simulink model "Scratch3"  (Simulink 8.5)
settings: Solver=ode4  StartTime=0.0  StopTime=20  FixedStep=0.005  RelTol=1e-3
model workspace (MAT data in the model file):
  Jm1 = 0.9333
  Jm2 = 0.6533
  Jm3 = 0.6533
  Jm4 = 0.4667
  k1 = 100
  k2 = 100
  k3 = 100
  k4 = 100
  Fv1 = 15
  Fv2 = 12
  Fv3 = 1
  Fv4 = 1
  Kp1 = 15
  Kp2 = 20
  Kp3 = 5
  Kp4 = 5
  Kd1 = 5
  Kd2 = 10
  Kd3 = 2
  Kd4 : num (value not decoded)
libraries: dspinverses x1, roblocks x1
(part 1 of 3)
settings Model: Creator=ahmad  LastModifiedBy=ahmad
settings DataIOCC: SignalLoggingSaveFormat=Dataset
settings OptimizationCC: ExpressionDepthLimit=128
settings DebuggingCC: UnderspecifiedInitializationDetection=Simplified  MergeDetectMultiDrivingBlocksExec=error  FcnCallInpInsideContextMsg=EnableAllAsError  StateNameClashWarn=none
settings GRTTargetCC: CombineOutputUpdateFcns=on  GRTInterface=off

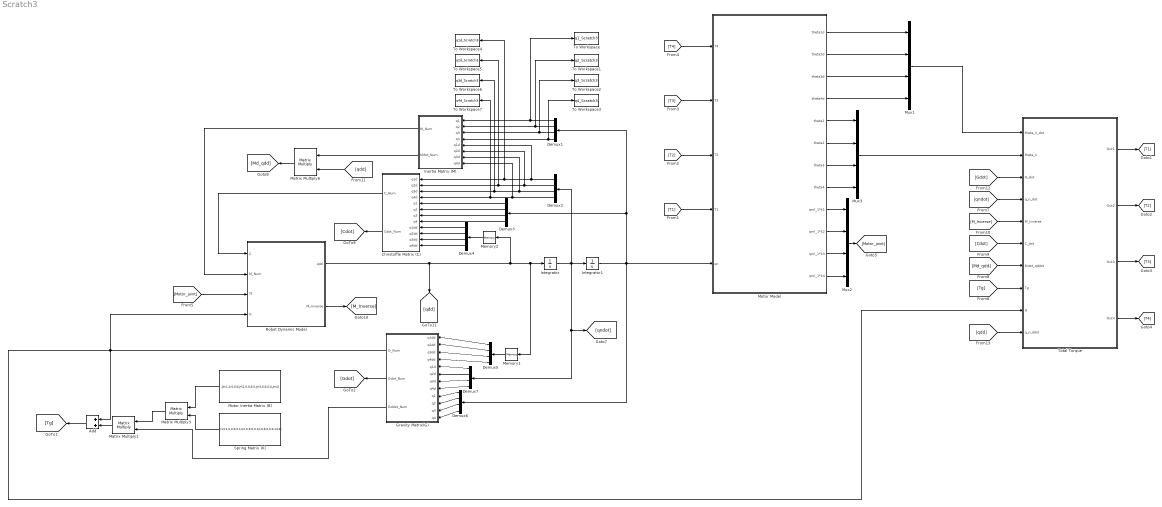
== system Scratch3 ==
  Add : Sum
  Christoffle Matrix (C) : MATLAB Function  TreatAsAtomicUnit=on
  Demux{1..7} (7 alike) : Demux
  Gravity Matrix(G) : MATLAB Function  TreatAsAtomicUnit=on
  Inertia Matrix (M) : MATLAB Function  TreatAsAtomicUnit=on
  Integrator : Integrator
  Integrator1 : Integrator
  Matrix Multiply1 : Product  Multiplication=Matrix(*)
  Matrix Multiply3 : Product  Multiplication=Matrix(*)
  Matrix Multiply6 : Product  Multiplication=Matrix(*)
  Memory1 : Memory
  Memory2 : Memory
  Motor Inertia Matrix (B) : Constant  Value=[Jm1,0,0,0;0,Jm2,0,0;0,0,Jm3,0;0,0,0,Jm4]  VectorParams1D=off
  "Motor Model " : Subsystem
  Mux1 : Mux
  Mux2 : Mux
  Mux3 : Mux
  "Robot Dynamic Model " : MATLAB Function  TreatAsAtomicUnit=on
  Spring Matrix (K) : Constant  Value=[1/k1,0,0,0;0,1/k2,0,0;0,0,1/k3,0;0,0,0,1/k4]  VectorParams1D=off
  To Workspace : ToWorkspace  VariableName=q1_Scratch3  SaveFormat=Structure With Time  SampleTime=-1
  To Workspace1 : ToWorkspace  VariableName=q2_Scratch3  SaveFormat=Structure With Time  SampleTime=-1
  To Workspace2 : ToWorkspace  VariableName=q3_Scratch3  SaveFormat=Structure With Time  SampleTime=-1
  To Workspace3 : ToWorkspace  VariableName=q4_Scratch3  SaveFormat=Structure With Time  SampleTime=-1
  To Workspace4 : ToWorkspace  VariableName=q1d_Scratch3  SaveFormat=Structure With Time  SampleTime=-1
  To Workspace5 : ToWorkspace  VariableName=q2d_Scratch3  SaveFormat=Structure With Time  SampleTime=-1
  To Workspace6 : ToWorkspace  VariableName=q3d_Scratch3  SaveFormat=Structure With Time  SampleTime=-1
  To Workspace7 : ToWorkspace  VariableName=q4d_Scratch3  SaveFormat=Structure With Time  SampleTime=-1
  "Total Torque " : Subsystem
  wires:
  [T1] -> "Motor Model "/4(T1)
  [T2] -> "Motor Model "/3(T2)
  [T3] -> "Motor Model "/2(T3)
  [T4] -> "Motor Model "/1(T4)
  "Motor Model "/9(qml_1*k1) -> Mux2/1
  "Motor Model "/10(qml_1*k2) -> Mux2/2
  "Motor Model "/11(qml_1*k3) -> Mux2/3
  "Motor Model "/12(qml_1*k4) -> Mux2/4
  Mux2/1 -> [Motor_joint]
  "Total Torque "/4(Out4) -> [T4]
  "Total Torque "/3(Out3) -> [T3]
  "Total Torque "/2(Out2) -> [T2]
  "Total Torque "/1(Out1) -> [T1]
  "Motor Model "/1(theta1d) -> Mux1/1
  "Motor Model "/2(theta2d) -> Mux1/2
  "Motor Model "/3(theta3d) -> Mux1/3
  "Motor Model "/4(theta4d) -> Mux1/4
  Integrator/1 -> Demux7/1, [qndot], Demux2/1, Integrator1/1
  Integrator1/1 -> Demux1/1, Demux3/1, "Motor Model "/5(qn), Demux6/1
  Demux2/1 -> Inertia Matrix (M)/5(q1d), To Workspace4/1, Christoffle Matrix (C)/1(q1d)
  Demux2/2 -> Inertia Matrix (M)/6(q2d), To Workspace5/1, Christoffle Matrix (C)/2(q2d)
  Demux2/3 -> Inertia Matrix (M)/7(q3d), To Workspace6/1, Christoffle Matrix (C)/3(q3d)
  Demux2/4 -> Inertia Matrix (M)/8(q4d), Christoffle Matrix (C)/4(q4d), To Workspace7/1
  Demux3/1 -> Christoffle Matrix (C)/5(q1)
  Demux3/2 -> Christoffle Matrix (C)/6(q2)
  Demux3/3 -> Christoffle Matrix (C)/7(q3)
  Demux3/4 -> Christoffle Matrix (C)/8(q4)
  Demux1/1 -> Inertia Matrix (M)/1(q1), To Workspace/1
  Demux1/2 -> Inertia Matrix (M)/2(q2), To Workspace1/1
  Demux1/3 -> Inertia Matrix (M)/3(q3), To Workspace2/1
  Demux1/4 -> Inertia Matrix (M)/4(q4), To Workspace3/1
  Demux4/1 -> Christoffle Matrix (C)/9(q1dd)
  Demux4/2 -> Christoffle Matrix (C)/10(q2dd)
  Demux4/3 -> Christoffle Matrix (C)/11(q3dd)
  Demux4/4 -> Christoffle Matrix (C)/12(q4dd)
  Christoffle Matrix (C)/2(Cdot_Num) -> [Cdot]
  [qdd] -> Matrix Multiply6/2
  Matrix Multiply6/1 -> [Md_qdd]
  "Robot Dynamic Model "/2(M_Inverse) -> [M_Inverse]
  [M_Inverse] -> "Total Torque "/5(M_Inverse)
  [Md_qdd] -> "Total Torque "/7(Mdot_qddot)
  [Cdot] -> "Total Torque "/6(C_dot)
  [qndot] -> "Total Torque "/4(q_n_dot)
  "Robot Dynamic Model "/1(qdd) -> [qdd], Memory1/1, Integrator/1, Memory2/1
  Inertia Matrix (M)/2(Mdot_Num) -> Matrix Multiply6/1
  [Tg] -> "Total Torque "/8(Tg)
  Motor Inertia Matrix (B)/1 -> Matrix Multiply3/1
  Spring Matrix (K)/1 -> Matrix Multiply3/2
  Matrix Multiply3/1 -> Matrix Multiply1/1
  Demux6/1 -> Gravity Matrix(G)/9(q1)
  Demux6/2 -> Gravity Matrix(G)/10(q2)
  Demux6/3 -> Gravity Matrix(G)/11(q3)
  Demux6/4 -> Gravity Matrix(G)/12(q4)
  Demux5/1 -> Gravity Matrix(G)/1(q1dd)
  Demux5/2 -> Gravity Matrix(G)/2(q2dd)
  Demux5/3 -> Gravity Matrix(G)/3(q3dd)
  Demux5/4 -> Gravity Matrix(G)/4(q4dd)
  Demux7/1 -> Gravity Matrix(G)/5(q1d)
  Demux7/2 -> Gravity Matrix(G)/6(q2d)
  Demux7/3 -> Gravity Matrix(G)/7(q3d)
  Demux7/4 -> Gravity Matrix(G)/8(q4d)
  Add/1 -> [Tg]
  Matrix Multiply1/1 -> Add/2
  [Gdot] -> "Total Torque "/3(G_dot)
  "Motor Model "/8(theta4) -> Mux3/4
  "Motor Model "/7(theta3) -> Mux3/3
  "Motor Model "/6(theta2) -> Mux3/2
  "Motor Model "/5(theta1) -> Mux3/1
  Mux3/1 -> "Total Torque "/2(theta_n)
  Mux1/1 -> "Total Torque "/1(theta_n_dot)
  Christoffle Matrix (C)/1(C_Num) -> "Robot Dynamic Model "/1(C)
  [Motor_joint] -> "Robot Dynamic Model "/3(Tf)
  Inertia Matrix (M)/1(M_Num) -> "Robot Dynamic Model "/2(M_Num)
  [qdd] -> "Total Torque "/10("q_n_ddot ")
  Gravity Matrix(G)/1(G_Num) -> "Robot Dynamic Model "/4(G), "Total Torque "/9(G), Add/1
  Memory2/1 -> Demux4/1
  Memory1/1 -> Demux5/1
  Gravity Matrix(G)/3(Gddot_Num) -> Matrix Multiply1/2
  Gravity Matrix(G)/2(Gdot_Num) -> [Gdot]

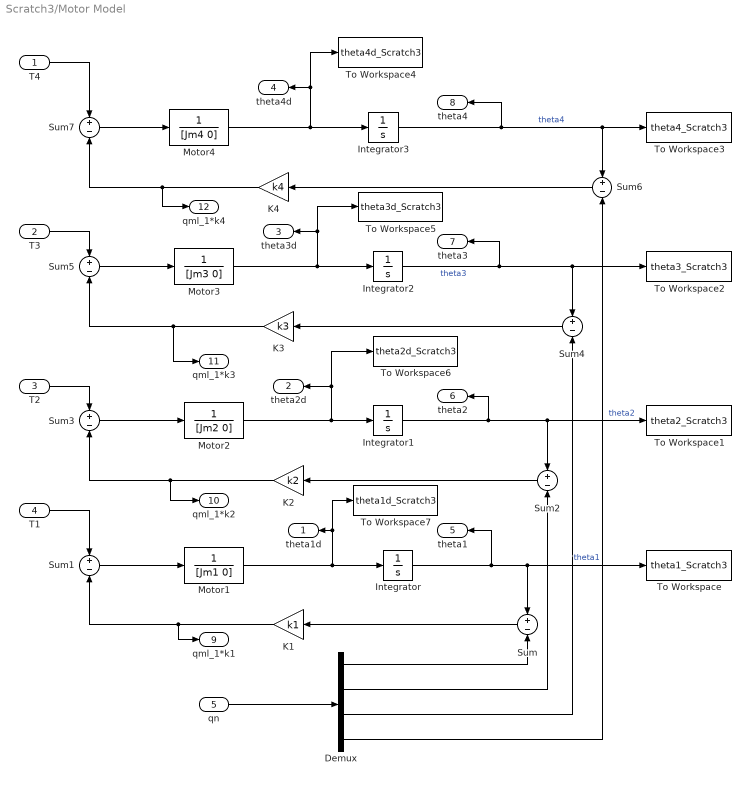
== system Scratch3/Motor Model  ==
  T4 : Inport
  T3 : Inport  Port=2
  T2 : Inport  Port=3
  T1 : Inport  Port=4
  qn : Inport  Port=5
  "\tK1 " : Gain  Gain=k1
  "\tK2 " : Gain  Gain=k2
  "\tK3 " : Gain  Gain=k3
  "\tK4 " : Gain  Gain=k4
  Demux : Demux
  Integrator{,1..3} (4 alike) : Integrator
  Motor1 : TransferFcn  Denominator=[Jm1 0]
  Motor2 : TransferFcn  Denominator=[Jm2 0]
  Motor3 : TransferFcn  Denominator=[Jm3 0]
  Motor4 : TransferFcn  Denominator=[Jm4 0]
  Sum{,1..7} (8 alike) : Sum  Inputs=+-
  To Workspace : ToWorkspace  VariableName=theta1_Scratch3  SaveFormat=Structure With Time  SampleTime=-1
  To Workspace1 : ToWorkspace  VariableName=theta2_Scratch3  SaveFormat=Structure With Time  SampleTime=-1
  To Workspace2 : ToWorkspace  VariableName=theta3_Scratch3  SaveFormat=Structure With Time  SampleTime=-1
  To Workspace3 : ToWorkspace  VariableName=theta4_Scratch3  SaveFormat=Structure With Time  SampleTime=-1
  To Workspace4 : ToWorkspace  VariableName=theta4d_Scratch3  SaveFormat=Structure With Time  SampleTime=-1
  To Workspace5 : ToWorkspace  VariableName=theta3d_Scratch3  SaveFormat=Structure With Time  SampleTime=-1
  To Workspace6 : ToWorkspace  VariableName=theta2d_Scratch3  SaveFormat=Structure With Time  SampleTime=-1
  To Workspace7 : ToWorkspace  VariableName=theta1d_Scratch3  SaveFormat=Structure With Time  SampleTime=-1
  theta1d : Outport
  theta2d : Outport  Port=2
  theta3d : Outport  Port=3
  theta4d : Outport  Port=4
  theta1 : Outport  Port=5
  theta2 : Outport  Port=6
  theta3 : Outport  Port=7
  theta4 : Outport  Port=8
  qml_1*k1 : Outport  Port=9
  qml_1*k2 : Outport  Port=10
  qml_1*k3 : Outport  Port=11
  qml_1*k4 : Outport  Port=12
  wires:
  qn/1 -> Demux/1
  Demux/1 -> Sum/2
  Motor1/1 -> Integrator/1, To Workspace7/1, theta1d/1
  Integrator/1 -> theta1/1, To Workspace/1, Sum/1  "theta1"
  Sum/1 -> "\tK1 "/1
  "\tK1 "/1 -> Sum1/2, qml_1*k1/1
  Sum1/1 -> Motor1/1
  Motor2/1 -> To Workspace6/1, theta2d/1, Integrator1/1
  Integrator1/1 -> theta2/1, To Workspace1/1, Sum2/1  "theta2"
  Sum2/1 -> "\tK2 "/1
  "\tK2 "/1 -> qml_1*k2/1, Sum3/2
  Sum3/1 -> Motor2/1
  Demux/2 -> Sum2/2
  Motor3/1 -> To Workspace5/1, theta3d/1, Integrator2/1
  Integrator2/1 -> theta3/1, To Workspace2/1, Sum4/1  "theta3"
  Sum4/1 -> "\tK3 "/1
  "\tK3 "/1 -> qml_1*k3/1, Sum5/2
  Sum5/1 -> Motor3/1
  Demux/3 -> Sum4/2
  Motor4/1 -> To Workspace4/1, theta4d/1, Integrator3/1
  Integrator3/1 -> theta4/1, To Workspace3/1, Sum6/1  "theta4"
  Sum6/1 -> "\tK4 "/1
  "\tK4 "/1 -> qml_1*k4/1, Sum7/2
  Sum7/1 -> Motor4/1
  Demux/4 -> Sum6/2
  T4/1 -> Sum7/1
  T3/1 -> Sum5/1
  T2/1 -> Sum3/1
  T1/1 -> Sum1/1

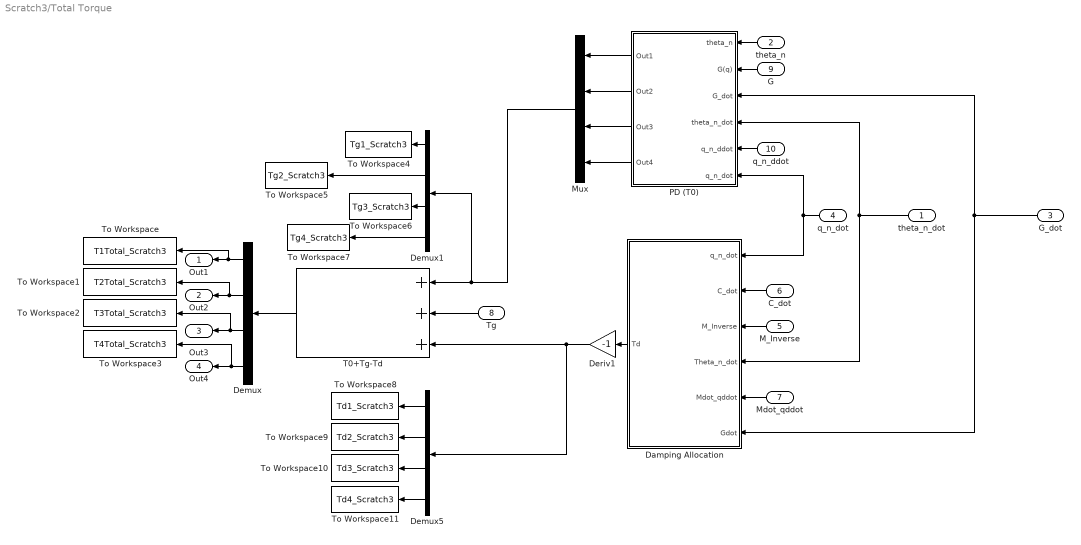
== system Scratch3/Total Torque  ==
  theta_n_dot : Inport
  theta_n : Inport  Port=2
  G_dot : Inport  Port=3
  q_n_dot : Inport  Port=4
  M_Inverse : Inport  Port=5
  C_dot : Inport  Port=6
  Mdot_qddot : Inport  Port=7
  Tg : Inport  Port=8
  G : Inport  Port=9
  "q_n_ddot " : Inport  Port=10
  Damping Allocation : Subsystem
  Demux : Demux
  Demux1 : Demux
  Demux5 : Demux
  Deriv1 : Gain  Gain=-1
  Mux : Mux
  PD (T0) : Subsystem
  T0+Tg-Td : Sum  Inputs=+++
  To Workspace : ToWorkspace  VariableName=T1Total_Scratch3  SaveFormat=Structure With Time  SampleTime=-1
  To Workspace1 : ToWorkspace  VariableName=T2Total_Scratch3  SaveFormat=Structure With Time  SampleTime=-1
  To Workspace10 : ToWorkspace  VariableName=Td3_Scratch3  SaveFormat=Structure With Time  SampleTime=-1
  To Workspace11 : ToWorkspace  VariableName=Td4_Scratch3  SaveFormat=Structure With Time  SampleTime=-1
  To Workspace2 : ToWorkspace  VariableName=T3Total_Scratch3  SaveFormat=Structure With Time  SampleTime=-1
  To Workspace3 : ToWorkspace  VariableName=T4Total_Scratch3  SaveFormat=Structure With Time  SampleTime=-1
  To Workspace4 : ToWorkspace  VariableName=Tg1_Scratch3  SaveFormat=Structure With Time  SampleTime=-1
  To Workspace5 : ToWorkspace  VariableName=Tg2_Scratch3  SaveFormat=Structure With Time  SampleTime=-1
  To Workspace6 : ToWorkspace  VariableName=Tg3_Scratch3  SaveFormat=Structure With Time  SampleTime=-1
  To Workspace7 : ToWorkspace  VariableName=Tg4_Scratch3  SaveFormat=Structure With Time  SampleTime=-1
  To Workspace8 : ToWorkspace  VariableName=Td1_Scratch3  SaveFormat=Structure With Time  SampleTime=-1
  To Workspace9 : ToWorkspace  VariableName=Td2_Scratch3  SaveFormat=Structure With Time  SampleTime=-1
  Out1 : Outport
  Out2 : Outport  Port=2
  Out3 : Outport  Port=3
  Out4 : Outport  Port=4
  wires:
  PD (T0)/1(Out1) -> Mux/1
  PD (T0)/2(Out2) -> Mux/2
  PD (T0)/3(Out3) -> Mux/3
  PD (T0)/4(Out4) -> Mux/4
  T0+Tg-Td/1 -> Demux/1
  Demux/2 -> To Workspace1/1, Out2/1
  Demux/3 -> To Workspace2/1, Out3/1
  Demux/4 -> To Workspace3/1, Out4/1
  Tg/1 -> T0+Tg-Td/2
  Damping Allocation/1(Td) -> Deriv1/1
  C_dot/1 -> Damping Allocation/2(C_dot)
  M_Inverse/1 -> Damping Allocation/3(M_Inverse)
  q_n_dot/1 -> Damping Allocation/1(q_n_dot), PD (T0)/6(q_n_dot)
  Mdot_qddot/1 -> Damping Allocation/5(Mdot_qddot)
  G_dot/1 -> Damping Allocation/6(Gdot), PD (T0)/3("G_dot ")
  theta_n/1 -> PD (T0)/1(theta_n)
  G/1 -> PD (T0)/2("G(q) ")
  Mux/1 -> Demux1/1, T0+Tg-Td/1
  "q_n_ddot "/1 -> PD (T0)/5(q_n_ddot)
  theta_n_dot/1 -> PD (T0)/4(theta_n_dot), Damping Allocation/4(Theta_n_dot)
  Demux/1 -> To Workspace/1, Out1/1
  Demux1/2 -> To Workspace5/1
  Demux1/1 -> To Workspace4/1
  Demux1/3 -> To Workspace6/1
  Demux1/4 -> To Workspace7/1
  Demux5/1 -> To Workspace8/1
  Demux5/2 -> To Workspace9/1
  Demux5/3 -> To Workspace10/1
  Demux5/4 -> To Workspace11/1
  Deriv1/1 -> Demux5/1, T0+Tg-Td/3

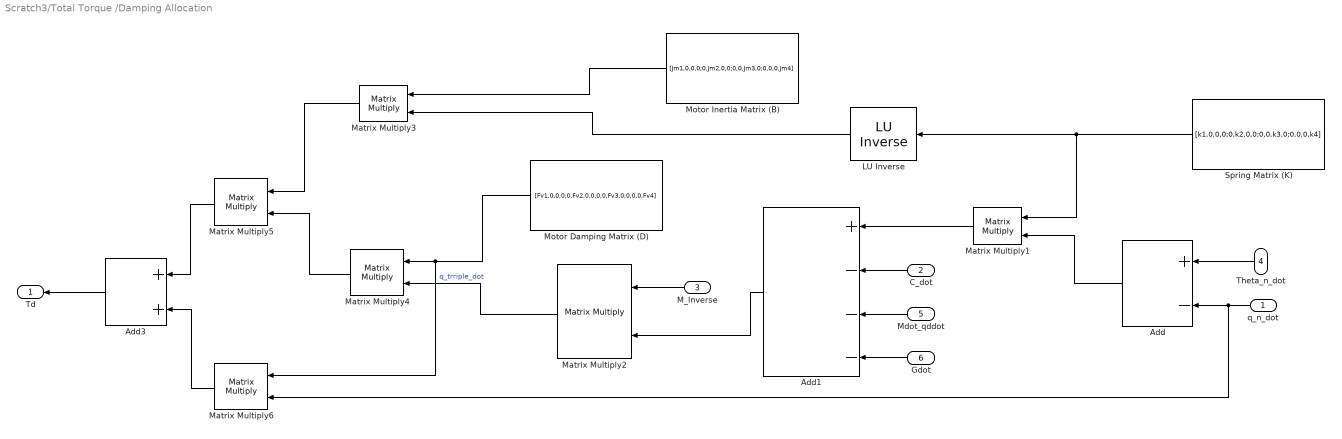
== system Scratch3/Total Torque /Damping Allocation ==
  q_n_dot : Inport
  C_dot : Inport  Port=2
  M_Inverse : Inport  Port=3
  Theta_n_dot : Inport  Port=4
  Mdot_qddot : Inport  Port=5
  Gdot : Inport  Port=6
  " LU Inverse" : dspinverses/ LU Inverse
  Add : Sum  Inputs=+-
  Add1 : Sum  Inputs=+---
  Add3 : Sum
  Matrix Multiply{1..6} (6 alike) : Product  Multiplication=Matrix(*)
  Motor Damping Matrix (D) : Constant  Value=[Fv1,0,0,0;0,Fv2,0,0;0,0,Fv3,0;0,0,0,Fv4]  VectorParams1D=off
  Motor Inertia Matrix (B) : Constant  Value=[Jm1,0,0,0;0,Jm2,0,0;0,0,Jm3,0;0,0,0,Jm4]  VectorParams1D=off
  Spring Matrix (K) : Constant  Value=[k1,0,0,0;0,k2,0,0;0,0,k3,0;0,0,0,k4]  VectorParams1D=off
  Td : Outport
  wires:
  Matrix Multiply5/1 -> Add3/1
  Matrix Multiply6/1 -> Add3/2
  q_n_dot/1 -> Matrix Multiply6/2, Add/2
  Spring Matrix (K)/1 -> Matrix Multiply1/1, " LU Inverse"/1
  Add/1 -> Matrix Multiply1/2
  Matrix Multiply1/1 -> Add1/1
  Add1/1 -> Matrix Multiply2/2
  Matrix Multiply2/1 -> Matrix Multiply4/2  "q_trriple_dot"
  Matrix Multiply4/1 -> Matrix Multiply5/2
  Motor Inertia Matrix (B)/1 -> Matrix Multiply3/1
  " LU Inverse"/1 -> Matrix Multiply3/2
  Motor Damping Matrix (D)/1 -> Matrix Multiply6/1, Matrix Multiply4/1
  Matrix Multiply3/1 -> Matrix Multiply5/1
  M_Inverse/1 -> Matrix Multiply2/1
  C_dot/1 -> Add1/2
  Mdot_qddot/1 -> Add1/3
  Add3/1 -> Td/1
  Theta_n_dot/1 -> Add/1
  Gdot/1 -> Add1/4

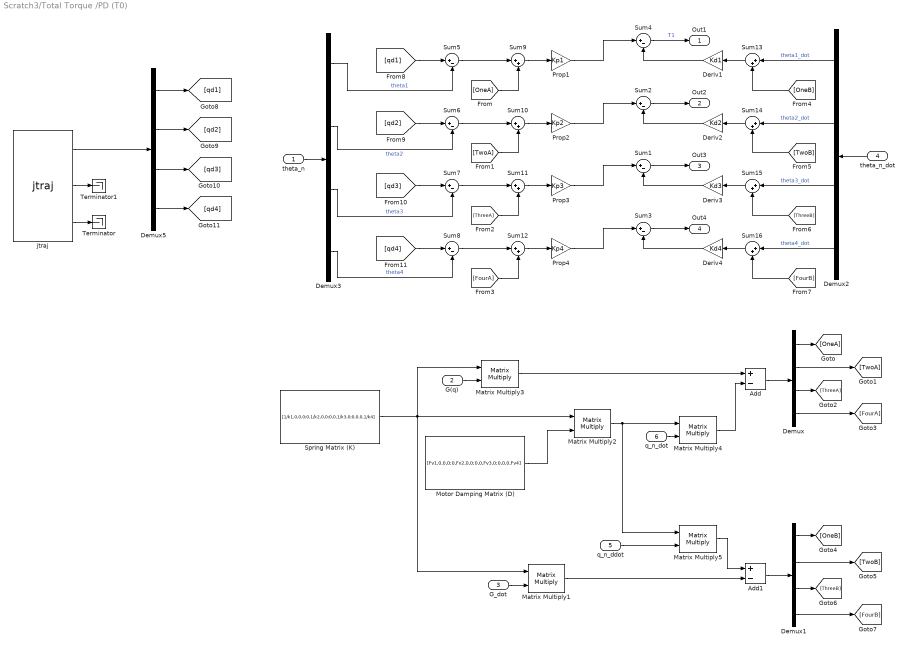
== system Scratch3/Total Torque /PD (T0) ==
  theta_n : Inport
  "G(q) " : Inport  Port=2
  "G_dot " : Inport  Port=3
  theta_n_dot : Inport  Port=4
  q_n_ddot : Inport  Port=5
  q_n_dot : Inport  Port=6
  Add : Sum  Inputs=+-
  Add1 : Sum  Inputs=+-
  Demux{,1..3,5} (5 alike) : Demux
  Deriv1 : Gain  Gain=Kd1
  Deriv2 : Gain  Gain=Kd2
  Deriv3 : Gain  Gain=Kd3
  Deriv4 : Gain  Gain=Kd4
  Matrix Multiply{1..5} (5 alike) : Product  Multiplication=Matrix(*)
  Motor Damping Matrix (D) : Constant  Value=[Fv1,0,0,0;0,Fv2,0,0;0,0,Fv3,0;0,0,0,Fv4]  VectorParams1D=off
  Prop1 : Gain  Gain=Kp1
  Prop2 : Gain  Gain=Kp2
  Prop3 : Gain  Gain=Kp3
  Prop4 : Gain  Gain=Kp4
  Spring Matrix (K) : Constant  Value=[1/k1,0,0,0;0,1/k2,0,0;0,0,1/k3,0;0,0,0,1/k4]  VectorParams1D=off
  Sum{1..8} (8 alike) : Sum  Inputs=|+-  SaturateOnIntegerOverflow=on  InputSameDT=on  OutDataTypeStr=Inherit: Same as first input
  Sum{9..16} (8 alike) : Sum  Inputs=|++  SaturateOnIntegerOverflow=on  InputSameDT=on  OutDataTypeStr=Inherit: Same as first input
  Terminator : Terminator
  Terminator1 : Terminator
  jtraj : roblocks/Trajectory/jtraj  q0=[0 0 0 0]  qf=[pi/2 -pi/2 pi/4 3*pi/2]  tmax=20  ts=0.005
  Out1 : Outport
  Out2 : Outport  Port=2
  Out3 : Outport  Port=3
  Out4 : Outport  Port=4
  wires:
  Sum4/1 -> Out1/1  "T1"
  Demux3/4 -> Sum8/2  "theta4"
  Demux2/2 -> Sum14/1  "theta2_dot"
  Demux2/3 -> Sum15/1  "theta3_dot"
  Demux2/4 -> Sum16/1  "theta4_dot"
  Demux2/1 -> Sum13/1  "theta1_dot"
  Sum3/1 -> Out4/1
  Sum1/1 -> Out3/1
  Sum2/1 -> Out2/1
  theta_n_dot/1 -> Demux2/1
  theta_n/1 -> Demux3/1
  Demux3/1 -> Sum5/2  "theta1"
  Demux3/2 -> Sum6/2  "theta2"
  Demux3/3 -> Sum7/2  "theta3"
  Sum9/1 -> Prop1/1
  Sum11/1 -> Prop3/1
  Sum12/1 -> Prop4/1
  Sum10/1 -> Prop2/1
  Spring Matrix (K)/1 -> Matrix Multiply2/1, Matrix Multiply1/1, Matrix Multiply3/1
  "G_dot "/1 -> Matrix Multiply1/2
  "G(q) "/1 -> Matrix Multiply3/2
  Sum5/1 -> Sum9/1
  [OneA] -> Sum9/2
  Sum6/1 -> Sum10/1
  Sum7/1 -> Sum11/1
  Sum8/1 -> Sum12/1
  [TwoA] -> Sum10/2
  [ThreeA] -> Sum11/2
  [FourA] -> Sum12/2
  [OneB] -> Sum13/2
  [TwoB] -> Sum14/2
  [ThreeB] -> Sum15/2
  [FourB] -> Sum16/2
  Sum16/1 -> Deriv4/1
  Sum15/1 -> Deriv3/1
  Sum14/1 -> Deriv2/1
  Sum13/1 -> Deriv1/1
  Deriv1/1 -> Sum4/2
  Deriv2/1 -> Sum2/2
  Deriv3/1 -> Sum1/2
  Deriv4/1 -> Sum3/2
  Prop4/1 -> Sum3/1
  Prop3/1 -> Sum1/1
  Prop2/1 -> Sum2/1
  Prop1/1 -> Sum4/1
  Add/1 -> Demux/1
  Demux/1 -> [OneA]
  Demux/3 -> [ThreeA]
  Demux/2 -> [TwoA]
  Demux/4 -> [FourA]
  Matrix Multiply3/1 -> Add/1
  Motor Damping Matrix (D)/1 -> Matrix Multiply2/2
  Matrix Multiply2/1 -> Matrix Multiply4/1, Matrix Multiply5/1
  q_n_dot/1 -> Matrix Multiply4/2
  Matrix Multiply4/1 -> Add/2
  Add1/1 -> Demux1/1
  Demux1/1 -> [OneB]
  Demux1/2 -> [TwoB]
  Demux1/3 -> [ThreeB]
  Demux1/4 -> [FourB]
  Matrix Multiply1/1 -> Add1/2
  q_n_ddot/1 -> Matrix Multiply5/2
  Matrix Multiply5/1 -> Add1/1
  jtraj/3 -> Terminator/1
  jtraj/2 -> Terminator1/1
  jtraj/1 -> Demux5/1
  Demux5/1 -> [qd1]
  Demux5/2 -> [qd2]
  Demux5/3 -> [qd3]
  Demux5/4 -> [qd4]
  [qd1] -> Sum5/1
  [qd2] -> Sum6/1
  [qd3] -> Sum7/1
  [qd4] -> Sum8/1

== matlab function Inertia Matrix (M) ==
  data: M_Num output double; Mdot_Num output double; q1 input double; q2 input double; q3 input double; q4 input double; q1d input double; q2d input double; q3d input double; q4d input double
function [M_Num,Mdot_Num]  = fcn(q1, q2, q3, q4, q1d, q2d, q3d, q4d)
%#codegen
% coder.extrinsic('evalin'); 
% coder.extrinsic('subs'); 
% coder.extrinsic('eval'); 
% 
% qsym = evalin('base','q');
% Msym = evalin('base','M');
% StatesSym = evalin('base','states1');
% MdotSym = evalin('base','Mdot');
% 
% q_Num= [q1t;q2t;q3t;q4t];
% States_Num = [q1t;q2t;q3t;q4t;q1dt;q2dt;q3dt;q4dt];
% 
% M_Num = zeros(4,4);
% Mdot_Num = zeros(4,4);
% 
% M_Num = eval(subs(Msym,qsym,q_Num));
% Mdot_Num = eval(subs(MdotSym,StatesSym,States_Num));

m1 = 10;
m2 = 7;
m3 = 7;
m4 = 5;
l1 = 1;
l2 = 0.7;
l3 = 0.7; 
l4 = 0.5;
d1 = l1/2;
d2 = l2/2;
d3 = l3/2; 
d4 = l4/2;
I1zz = 0.9333;
I2zz = 0.6533;
I3zz = 0.6533;
I4zz = 0.4667;

M_Num = [I1zz + I2zz + I3zz + I4zz + d1^2*m1 + (d2^2*m2)/2 + d3^2*m3 + d4^2*m4 + (l1^2*m2)/2 + l1^2*m3 + l1^2*m4 + l2^2*m3 + l2^2*m4 + l3^2*m4 - (l1^2*m2*cos(2*q1))/2 - (d2^2*m2*cos(2*q1 + 2*q2))/2 + 2*d3*l1*m3*cos(q2 + q3) + 2*d4*l2*m4*cos(q3 + q4) + 2*l1*l3*m4*cos(q2 + q3) + d2*l1*m2*cos(q2) + 2*d3*l2*m3*cos(q3) + 2*d4*l3*m4*cos(q4) + 2*l1*l2*m3*cos(q2) + 2*l1*l2*m4*cos(q2) + 2*l2*l3*m4*cos(q3) - d2*l1*m2*cos(2*q1 + q2) + 2*d4*l1*m4*cos(q2 + q3 + q4), I2zz + I3zz + I4zz + (d2^2*m2)/2 + d3^2*m3 + d4^2*m4 + l2^2*m3 + l2^2*m4 + l3^2*m4 - (d2^2*m2*cos(2*q1 + 2*q2))/2 + d3*l1*m3*cos(q2 + q3) + 2*d4*l2*m4*cos(q3 + q4) + l1*l3*m4*cos(q2 + q3) + (d2*l1*m2*cos(q2))/2 + 2*d3*l2*m3*cos(q3) + 2*d4*l3*m4*cos(q4) + l1*l2*m3*cos(q2) + l1*l2*m4*cos(q2) + 2*l2*l3*m4*cos(q3) - (d2*l1*m2*cos(2*q1 + q2))/2 + d4*l1*m4*cos(q2 + q3 + q4), I3zz + I4zz + d3^2*m3 + d4^2*m4 + l3^2*m4 + d3*l1*m3*cos(q2 + q3) + d4*l2*m4*cos(q3 + q4) + l1*l3*m4*cos(q2 + q3) + d3*l2*m3*cos(q3) + 2*d4*l3*m4*cos(q4) + l2*l3*m4*cos(q3) + d4*l1*m4*cos(q2 + q3 + q4), I4zz + d4^2*m4 + d4*l2*m4*cos(q3 + q4) + d4*l3*m4*cos(q4) + d4*l1*m4*cos(q2 + q3 + q4)
                                                                                      I2zz + I3zz + I4zz + (d2^2*m2)/2 + d3^2*m3 + d4^2*m4 + l2^2*m3 + l2^2*m4 + l3^2*m4 - (d2^2*m2*cos(2*q1 + 2*q2))/2 + d3*l1*m3*cos(q2 + q3) + 2*d4*l2*m4*cos(q3 + q4) + l1*l3*m4*cos(q2 + q3) + (d2*l1*m2*cos(q2))/2 + 2*d3*l2*m3*cos(q3) + 2*d4*l3*m4*cos(q4) + l1*l2*m3*cos(q2) + l1*l2*m4*cos(q2) + 2*l2*l3*m4*cos(q3) - (d2*l1*m2*cos(2*q1 + q2))/2 + d4*l1*m4*cos(q2 + q3 + q4),                                                                                                                                   I2zz + I3zz + I4zz + (d2^2*m2)/2 + d3^2*m3 + d4^2*m4 + (l1^2*m2)/2 + l2^2*m3 + l2^2*m4 + l3^2*m4 + (l1^2*m2*cos(2*q1))/2 - (d2^2*m2*cos(2*q1 + 2*q2))/2 + 2*d4*l2*m4*cos(q3 + q4) + 2*d3*l2*m3*cos(q3) + 2*d4*l3*m4*cos(q4) + 2*l2*l3*m4*cos(q3),                                                                              m3*d3^2 + l2*m3*cos(q3)*d3 + m4*d4^2 + 2*m4*cos(q4)*d4*l3 + l2*m4*cos(q3 + q4)*d4 + m4*l3^2 + l2*m4*cos(q3)*l3 + I3zz + I4zz,                              I4zz + d4^2*m4 + d4*l2*m4*cos(q3 + q4) + d4*l3*m4*cos(q4)
                                                                                                                                                                                                                                                               I3zz + I4zz + d3^2*m3 + d4^2*m4 + l3^2*m4 + d3*l1*m3*cos(q2 + q3) + d4*l2*m4*cos(q3 + q4) + l1*l3*m4*cos(q2 + q3) + d3*l2*m3*cos(q3) + 2*d4*l3*m4*cos(q4) + l2*l3*m4*cos(q3) + d4*l1*m4*cos(q2 + q3 + q4),                                                                                                                                                                                                                                                       m3*d3^2 + l2*m3*cos(q3)*d3 + m4*d4^2 + 2*m4*cos(q4)*d4*l3 + l2*m4*cos(q3 + q4)*d4 + m4*l3^2 + l2*m4*cos(q3)*l3 + I3zz + I4zz,                                                                                                                                            m3*d3^2 + m4*d4^2 + 2*m4*cos(q4)*d4*l3 + m4*l3^2 + I3zz + I4zz,                                                      m4*d4^2 + l3*m4*cos(q4)*d4 + I4zz
                                                                                                                                                                                                                                                                                                                                                                                  I4zz + d4^2*m4 + d4*l2*m4*cos(q3 + q4) + d4*l3*m4*cos(q4) + d4*l1*m4*cos(q2 + q3 + q4),                                                                                                                                                                                                                                                                                                                          I4zz + d4^2*m4 + d4*l2*m4*cos(q3 + q4) + d4*l3*m4*cos(q4),                                                                                                                                                                         m4*d4^2 + l3*m4*cos(q4)*d4 + I4zz,                                                                         m4*d4^2 + I4zz];
                                                                                                                                                                                                                                                                                                                                                                              
Mdot_Num = [q1d*(m2*sin(2*q1 + 2*q2)*d2^2 + 2*m2*sin(2*q1 + q2)*d2*l1 + m2*sin(2*q1)*l1^2) - q4d*(2*d4*l2*m4*sin(q3 + q4) + 2*d4*l3*m4*sin(q4) + 2*d4*l1*m4*sin(q2 + q3 + q4)) - q2d*(2*d3*l1*m3*sin(q2 + q3) - d2^2*m2*sin(2*q1 + 2*q2) + 2*l1*l3*m4*sin(q2 + q3) + d2*l1*m2*sin(q2) + 2*l1*l2*m3*sin(q2) + 2*l1*l2*m4*sin(q2) - d2*l1*m2*sin(2*q1 + q2) + 2*d4*l1*m4*sin(q2 + q3 + q4)) - q3d*(2*d3*l1*m3*sin(q2 + q3) + 2*d4*l2*m4*sin(q3 + q4) + 2*l1*l3*m4*sin(q2 + q3) + 2*d3*l2*m3*sin(q3) + 2*l2*l3*m4*sin(q3) + 2*d4*l1*m4*sin(q2 + q3 + q4)), q1d*(m2*sin(2*q1 + 2*q2)*d2^2 + l1*m2*sin(2*q1 + q2)*d2) - q2d*(d3*l1*m3*sin(q2 + q3) - d2^2*m2*sin(2*q1 + 2*q2) + l1*l3*m4*sin(q2 + q3) + (d2*l1*m2*sin(q2))/2 + l1*l2*m3*sin(q2) + l1*l2*m4*sin(q2) - (d2*l1*m2*sin(2*q1 + q2))/2 + d4*l1*m4*sin(q2 + q3 + q4)) - q4d*(2*d4*l2*m4*sin(q3 + q4) + 2*d4*l3*m4*sin(q4) + d4*l1*m4*sin(q2 + q3 + q4)) - q3d*(d3*l1*m3*sin(q2 + q3) + 2*d4*l2*m4*sin(q3 + q4) + l1*l3*m4*sin(q2 + q3) + 2*d3*l2*m3*sin(q3) + 2*l2*l3*m4*sin(q3) + d4*l1*m4*sin(q2 + q3 + q4)), - q2d*(d3*l1*m3*sin(q2 + q3) + l1*l3*m4*sin(q2 + q3) + d4*l1*m4*sin(q2 + q3 + q4)) - q4d*(d4*l2*m4*sin(q3 + q4) + 2*d4*l3*m4*sin(q4) + d4*l1*m4*sin(q2 + q3 + q4)) - q3d*(d3*l1*m3*sin(q2 + q3) + d4*l2*m4*sin(q3 + q4) + l1*l3*m4*sin(q2 + q3) + d3*l2*m3*sin(q3) + l2*l3*m4*sin(q3) + d4*l1*m4*sin(q2 + q3 + q4)), - q3d*(d4*l2*m4*sin(q3 + q4) + d4*l1*m4*sin(q2 + q3 + q4)) - q4d*(d4*l2*m4*sin(q3 + q4) + d4*l3*m4*sin(q4) + d4*l1*m4*sin(q2 + q3 + q4)) - d4*l1*m4*q2d*sin(q2 + q3 + q4)
                                 q1d*(m2*sin(2*q1 + 2*q2)*d2^2 + l1*m2*sin(2*q1 + q2)*d2) - q2d*(d3*l1*m3*sin(q2 + q3) - d2^2*m2*sin(2*q1 + 2*q2) + l1*l3*m4*sin(q2 + q3) + (d2*l1*m2*sin(q2))/2 + l1*l2*m3*sin(q2) + l1*l2*m4*sin(q2) - (d2*l1*m2*sin(2*q1 + q2))/2 + d4*l1*m4*sin(q2 + q3 + q4)) - q4d*(2*d4*l2*m4*sin(q3 + q4) + 2*d4*l3*m4*sin(q4) + d4*l1*m4*sin(q2 + q3 + q4)) - q3d*(d3*l1*m3*sin(q2 + q3) + 2*d4*l2*m4*sin(q3 + q4) + l1*l3*m4*sin(q2 + q3) + 2*d3*l2*m3*sin(q3) + 2*l2*l3*m4*sin(q3) + d4*l1*m4*sin(q2 + q3 + q4)),                                                                                                                                                                                                                                                                                           q1d*(m2*sin(2*q1 + 2*q2)*d2^2 - m2*sin(2*q1)*l1^2) - q4d*(2*d4*l2*m4*sin(q3 + q4) + 2*d4*l3*m4*sin(q4)) - q3d*(2*d4*l2*m4*sin(q3 + q4) + 2*d3*l2*m3*sin(q3) + 2*l2*l3*m4*sin(q3)) + d2^2*m2*q2d*sin(2*q1 + 2*q2),                                                                                                                                                                                              - q4d*(d4*l2*m4*sin(q3 + q4) + 2*d4*l3*m4*sin(q4)) - q3d*(d4*l2*m4*sin(q3 + q4) + d3*l2*m3*sin(q3) + l2*l3*m4*sin(q3)),                                                                                              - q4d*(d4*l2*m4*sin(q3 + q4) + d4*l3*m4*sin(q4)) - d4*l2*m4*q3d*sin(q3 + q4)
                                                                                                                                                                                                                        - q2d*(d3*l1*m3*sin(q2 + q3) + l1*l3*m4*sin(q2 + q3) + d4*l1*m4*sin(q2 + q3 + q4)) - q4d*(d4*l2*m4*sin(q3 + q4) + 2*d4*l3*m4*sin(q4) + d4*l1*m4*sin(q2 + q3 + q4)) - q3d*(d3*l1*m3*sin(q2 + q3) + d4*l2*m4*sin(q3 + q4) + l1*l3*m4*sin(q2 + q3) + d3*l2*m3*sin(q3) + l2*l3*m4*sin(q3) + d4*l1*m4*sin(q2 + q3 + q4)),                                                                                                                                                                                                                                                                                                                                                                                     - q4d*(d4*l2*m4*sin(q3 + q4) + 2*d4*l3*m4*sin(q4)) - q3d*(d4*l2*m4*sin(q3 + q4) + d3*l2*m3*sin(q3) + l2*l3*m4*sin(q3)),                                                                                                                                                                                                                                                                                             -2*d4*l3*m4*q4d*sin(q4),                                                                                                                                                     -d4*l3*m4*q4d*sin(q4)
                                                                                                                                                                                                                                                                                                                                                                  - q3d*(d4*l2*m4*sin(q3 + q4) + d4*l1*m4*sin(q2 + q3 + q4)) - q4d*(d4*l2*m4*sin(q3 + q4) + d4*l3*m4*sin(q4) + d4*l1*m4*sin(q2 + q3 + q4)) - d4*l1*m4*q2d*sin(q2 + q3 + q4),                                                                                                                                                                                                                                                                                                                                                                                                                               - q4d*(d4*l2*m4*sin(q3 + q4) + d4*l3*m4*sin(q4)) - d4*l2*m4*q3d*sin(q3 + q4),                                                                                                                                                                                                                                                                                               -d4*l3*m4*q4d*sin(q4),                                                                                                                                                                         0];

== matlab function Robot Dynamic Model  ==
  data: C input double; M_Num input double; Tf input double; qdd output double; M_Inverse output double; G input double
function [qdd, M_Inverse] = fcn(C, M_Num, Tf, G)
%#codegen
coder.extrinsic('simplify'); 

Torque = Tf-C-G;
M_Inverse = inv(M_Num);
qdd = M_Inverse*Torque;
